simulink model "ControlRealimentacionEstados"  (R2021b)
settings: Solver=VariableStepAuto  StartTime=0.0  StopTime=1000  RelTol=1e-3
values from neighbouring files (symbols this model uses):
  A_1 = eval(A)    [linealizacion.m]
  B_1 = eval(B)    [linealizacion.m]
  C = eye(2)    [linealizacion.m]
  GK = K    [linealizacion.m]
  K = place(A_1,B_1,[-50 -60])    [linealizacion.m]
  Ref = [16;15]    [linealizacion.m]
settings Model: Creator=Cesar  LastModifiedBy=Cesar

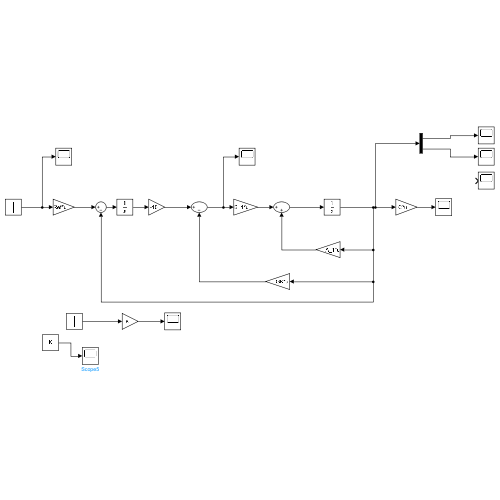
[thumbnail: Simulink's stored preview of the top-level diagram]
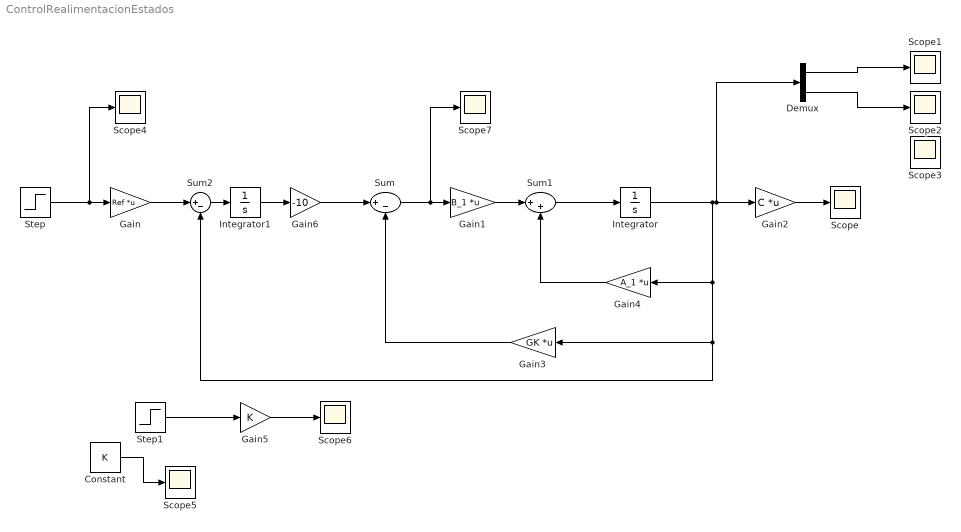
== system ControlRealimentacionEstados ==
  Constant : Constant  Value=K
  Demux : Demux  Outputs=2
  Gain : Gain  Gain=Ref  Multiplication=Matrix(K*u)
  Gain1 : Gain  Gain=B_1  Multiplication=Matrix(K*u)
  Gain2 : Gain  Gain=C  Multiplication=Matrix(K*u)
  Gain3 : Gain  Gain=GK  Multiplication=Matrix(K*u)
  Gain4 : Gain  Gain=A_1  Multiplication=Matrix(K*u)
  Gain5 : Gain  Gain=K
  Gain6 : Gain  Gain=-10
  Integrator : Integrator
  Integrator1 : Integrator
  Scope{,1..7} (8 alike) : Scope
  Step : Step  Time=0  SampleTime=0
  Step1 : Step  Time=0  SampleTime=0
  Sum : Sum  Inputs=|+-
  Sum1 : Sum  Inputs=|++
  Sum2 : Sum  Inputs=|+-
  wires:
  Gain4/1 -> Sum1/2
  Gain1/1 -> Sum1/1
  Sum/1 -> Scope7/1, Gain1/1
  Gain2/1 -> Scope/1
  Integrator/1 -> Gain4/1, Sum2/2, Gain3/1, Demux/1, Gain2/1
  Sum1/1 -> Integrator/1
  Gain3/1 -> Sum/2
  Step/1 -> Scope4/1, Gain/1
  Demux/1 -> Scope1/1
  Demux/2 -> Scope2/1
  Constant/1 -> Scope5/1
  Step1/1 -> Gain5/1
  Gain5/1 -> Scope6/1
  Sum2/1 -> Integrator1/1
  Gain/1 -> Sum2/1
  Integrator1/1 -> Gain6/1
  Gain6/1 -> Sum/1
